simulink model "full_model"  (R2021a)
settings: Solver=VariableStepAuto  StartTime=0.0  StopTime=50  RelTol=1e-3
values from neighbouring files (symbols this model uses):
  P = [real(P), imag(P)]    [black_pz.m]    (also in black_rlocus.m; black_rlocus_fine.m)
  R = rlocus(sys)    [black_rlocus.m]    (also in black_rlocus_fine.m = rlocus(sys,k))
undefined symbols (not defined in the file or in its folder): A_rocket, alpha_fine, Alt_sequence, Ang_max, Baro_exp, cm_fine, cm_lookup, Ct_rot, D, drag_lookup, drag_rot_lookup, drag_wave_lookup, g, h_0, I_s, I_x_lookup, I_yz_lookup, L_b, lift_lookup, lift_rot_lookup, m_burn, M_crit, M_fine, m_prop_max, m_wet, N, P_0, Phi, Pos_sequence, Psi, Q, r_E, S_e, T_b, T_lookup, T_max, T_max_s, t_P, t_S, t_V, Theta, Tilt_max, Ts_hev, Ts_hor, U, Upsilon, V, v_land, W
settings Model: Creator=EpEp  LastModifiedBy=EpEp
settings DebuggingCC: UnderSpecifiedDimensionMsg=warning

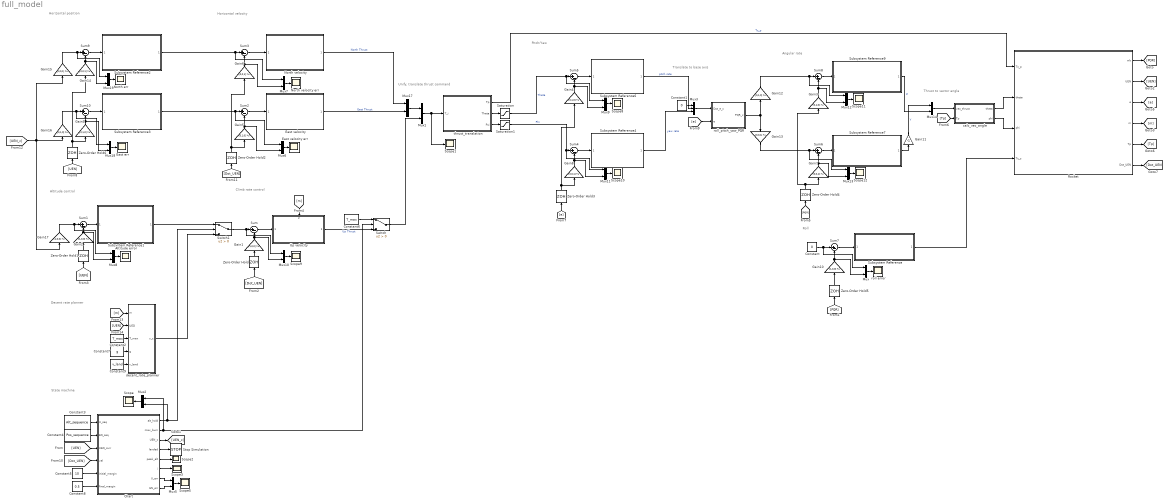
== system full_model ==
  note: Decent rate planner
  note: State machine
  note: Thrust to vector angle
  note: Roll
  note: Angular rate
  note: Translate to base axis
  note: Unify, translate thrust command
  note: Pitch/Yaw
  note: Climb rate control
  note: Altitude control
  note: Horizontal velocity
  note: Horizontal position
  Altitude error : Scope
  Chart : Stateflow chart  TreatAsAtomicUnit=on
  Constant : Constant  Value=0
  Constant1 : Constant  Value=0
  Constant2 : Constant  Value=T_max
  Constant3 : Constant  Value=Alt_sequence
  Constant4 : Constant  Value=Pos_sequence
  Constant5 : Constant  Value=10
  Constant6 : Constant  Value=T_max
  Constant7 : Constant  Value=g
  Constant8 : Constant  Value=0.5
  Constant9 : Constant  Value=v_land
  East err : Scope
  East velocity : Subsystem  ReferencedSubsystem=hor_vel_control
  East velocity err : Scope
  Gain{1..2,10,17} (4 alike) : Gain  Gain=[1,0,0]  Multiplication=Matrix(K*u)
  Gain11 : Gain  Gain=-1
  Gain{3..5,9,12,16} (6 alike) : Gain  Gain=[0,1,0]  Multiplication=Matrix(K*u)
  Gain{6..8,13..15} (6 alike) : Gain  Gain=[0,0,1]  Multiplication=Matrix(K*u)
  Mux{,1..2,5..14,17..19} (16 alike) : Mux  Inputs=2
  Mux3 : Mux  Inputs=3
  North err : Scope
  North velocity : Subsystem  ReferencedSubsystem=hor_vel_control
  North velocity err : Scope
  Rocket : Subsystem
  Saturation : Saturate  UpperLimit=Tilt_max  LowerLimit=-Tilt_max
  Saturation1 : Saturate  UpperLimit=Tilt_max  LowerLimit=-Tilt_max
  Scope{,1..3,5,8..12} (10 alike) : Scope
  Stop Simulation : Stop
  Subsystem Reference : Subsystem  ReferencedSubsystem=roll_controller
  Subsystem Reference1 : Subsystem  ReferencedSubsystem=alt_control
  Subsystem Reference2 : Subsystem  ReferencedSubsystem=pos_controller
  Subsystem Reference3 : Subsystem  ReferencedSubsystem=pos_controller
  Subsystem Reference4 : Subsystem  ReferencedSubsystem=ang_control
  Subsystem Reference6 : Subsystem  ReferencedSubsystem=ang_control
  Subsystem Reference7 : Subsystem  ReferencedSubsystem=rate_controller
  Subsystem Reference9 : Subsystem  ReferencedSubsystem=rate_controller
  Sum{,1..10} (11 alike) : Sum  Inputs=|+-
  Switch : Switch  Criteria=u2 > Threshold
  Switch1 : Switch  Criteria=u2 > Threshold
  Up velocity : Subsystem  ReferencedSubsystem=climb_control_PI
      settings: PortSchema="{\"entries\":[{\"content\":{\"sides\":[{\"content\":{\"connectorIds\":[\"In1\"]},\"type\":\"ConnectorPlacement.EquallySpacedRectSide\",\"uuid\":\"95254302-9a74-4c7f-a882-67c73735b286\"},{\"content\":{\"connectorIds\":[\"Out1\"],\"side\":\"RIGHT\"},\"type\":\"ConnectorPlacement.EquallySpacedRectSide\",\"uuid\":\"514a7716-605a-484c-b4b8-fcaa29f8a508\"},{\"content\":{\"connectorIds\":[\"In2\"],\"side\":\"TOP\"},\"type\":\"ConnectorPlacement.EquallySpacedRectSide\",\"uuid\":\"a977e3e4-e86d-439d-b6e9-39df081e30dd\"}]},\"type\":\"ConnectorPlacement.EquallySpacedConnector\",\"uuid\":\"b9474d80-c721-4f49-b50c-8544c213d6ea\"}],\"packageUris\":[\"http://schema.mathworks.com/mf0/Connector/R2020b\"],\"version\":\"1.0\"}"
  Zero-Order Hold : ZeroOrderHold  SampleTime=Ts_hev
  Zero-Order Hold1 : ZeroOrderHold  SampleTime=Ts_hev
  Zero-Order Hold{2..6} (5 alike) : ZeroOrderHold  SampleTime=Ts_hor
  calc_vec_angle : MATLAB Function  TreatAsAtomicUnit=on
  decent_rate_planner : MATLAB Function  TreatAsAtomicUnit=on
  roll error : Scope
  roll_pitch_yaw_PQR : MATLAB Function  TreatAsAtomicUnit=on
  thrust_translation : MATLAB Function  TreatAsAtomicUnit=on
  wires:
  Rocket/1(wb) -> [PQR]
  Rocket/2(UEN) -> [UEN]
  Gain1/1 -> Mux10/2, Sum/2
  [Dot_UEN] -> Zero-Order Hold/1
  Sum/1 -> Up velocity/1
  Sum1/1 -> Subsystem Reference1/1
  Gain2/1 -> Mux8/2, Sum1/2
  Rocket/4(m) -> [m]
  [m] -> Up velocity/2
  Subsystem Reference6/1 -> Mux3/2  "pitch rate"
  Sum8/1 -> Subsystem Reference9/1
  Gain3/1 -> Sum8/2, Mux12/2
  Rocket/3(e) -> [e]
  Gain4/1 -> Sum5/2, Mux9/2
  Sum5/1 -> Subsystem Reference6/1
  Sum2/1 -> East velocity/1
  Gain5/1 -> Sum2/2, Mux6/2
  Rocket/5(Tp) -> [Tp]
  East velocity/1 -> Mux17/2  "East Thrust"
  Zero-Order Hold2/1 -> Gain6/1, Gain5/1
  Sum3/1 -> North velocity/1
  Gain6/1 -> Mux7/2, Sum3/2
  North velocity/1 -> Mux17/1  "North Thrust"
  thrust_translation/1(Tp) -> Rocket/1(Tc_p)  "Tc_p"
  Subsystem Reference4/1 -> Mux3/3  "yaw rate"
  Gain8/1 -> Sum4/2, Mux11/2
  Gain7/1 -> Sum6/2, Mux13/2
  Sum4/1 -> Subsystem Reference4/1
  Sum6/1 -> Subsystem Reference7/1
  Zero-Order Hold4/1 -> Gain7/1, Gain3/1
  thrust_translation/2(Theta) -> Saturation/1
  thrust_translation/3(Psi) -> Saturation1/1
  Saturation/1 -> Sum5/1, Mux9/1  "Theta"
  Saturation1/1 -> Mux11/1, Sum4/1  "Phi"
  Subsystem Reference7/1 -> Gain11/1
  Zero-Order Hold/1 -> Gain1/1
  [UEN] -> Zero-Order Hold1/1
  Zero-Order Hold1/1 -> Gain2/1
  [Dot_UEN] -> Zero-Order Hold2/1
  [e] -> Zero-Order Hold3/1
  [PQR] -> Zero-Order Hold4/1
  Mux6/1 -> East velocity err/1
  Mux7/1 -> North velocity err/1
  Mux8/1 -> Altitude error/1
  Mux10/1 -> Scope9/1
  Mux9/1 -> Scope8/1
  Mux11/1 -> Scope10/1
  Mux12/1 -> Scope11/1
  Mux13/1 -> Scope12/1
  calc_vec_angle/2(phi) -> Rocket/3(phi)
  Mux1/1 -> Scope1/1, thrust_translation/1(T_i)
  Mux17/1 -> Mux1/1
  Subsystem Reference/1 -> Rocket/4(Tc_s)
  [PQR] -> Zero-Order Hold5/1
  Zero-Order Hold5/1 -> Gain10/1
  Gain10/1 -> Mux/2, Sum7/2
  Sum7/1 -> Subsystem Reference/1
  Constant/1 -> Mux/1, Sum7/1
  Mux/1 -> roll error/1
  calc_vec_angle/1(theta) -> Rocket/2(theta)
  Subsystem Reference9/1 -> Mux14/2  "Z"
  Gain11/1 -> Mux14/1  "Y"
  Mux14/1 -> calc_vec_angle/1(vec_thrust)
  [Tp] -> calc_vec_angle/2(Tp)
  Constant1/1 -> Mux3/1
  [e] -> roll_pitch_yaw_PQR/2(e)
  Mux3/1 -> roll_pitch_yaw_PQR/1(Dot_e_c)
  roll_pitch_yaw_PQR/1(PQR_c) -> Gain12/1, Gain13/1
  Gain12/1 -> Mux12/1, Sum8/1
  Gain13/1 -> Mux13/1, Sum6/1
  Constant3/1 -> Chart/1(U_seq)
  Constant4/1 -> Chart/2(EN_seq)
  Sum9/1 -> Subsystem Reference2/1
  Sum10/1 -> Subsystem Reference3/1
  Gain9/1 -> Mux18/2, Sum10/2
  [UEN] -> Zero-Order Hold6/1
  Zero-Order Hold6/1 -> Gain14/1, Gain9/1
  Gain14/1 -> Mux19/2, Sum9/2
  Mux18/1 -> East err/1
  Mux19/1 -> North err/1
  Zero-Order Hold3/1 -> Gain4/1, Gain8/1
  Rocket/6(Dot_UEN) -> [Dot_UEN]
  Subsystem Reference2/1 -> Mux7/1, Sum3/1
  Subsystem Reference3/1 -> Mux6/1, Sum2/1
  [UEN] -> Chart/3(UEN_curr)
  Constant5/1 -> Chart/5(initial_margin)
  Chart/4(landed) -> Stop Simulation/1
  Chart/1(alt_hold) -> Mux2/2, Switch1/2
  Switch1/1 -> Mux10/1, Sum/1
  Subsystem Reference1/1 -> Switch1/1
  Chart/2(max_burn) -> Mux2/1, Switch/2
  Mux2/1 -> Scope/1
  Constant6/1 -> Switch/1
  Switch/1 -> Mux1/2
  Up velocity/1 -> Switch/3  "Up Thrust"
  [Dot_UEN] -> Chart/4(vel)
  Chart/5(peak_alt) -> Scope2/1
  Constant8/1 -> Chart/6(final_margin)
  Chart/6(i) -> Scope3/1
  Chart/7(U_err) -> Mux5/1
  Chart/8(EN_err) -> Mux5/2
  Mux5/1 -> Scope5/1
  Chart/3(UEN_c) -> [UEN_c]
  Gain15/1 -> Mux19/1, Sum9/1
  Gain16/1 -> Mux18/1, Sum10/1
  [UEN_c] -> Gain17/1, Gain16/1, Gain15/1
  Gain17/1 -> Mux8/1, Sum1/1
  decent_rate_planner/1(v_c) -> Switch1/3
  [m] -> decent_rate_planner/1(m)
  Constant2/1 -> decent_rate_planner/3(T_max)
  Constant7/1 -> decent_rate_planner/4(g)
  Constant9/1 -> decent_rate_planner/5(v_land)
  [UEN] -> decent_rate_planner/2(UED)

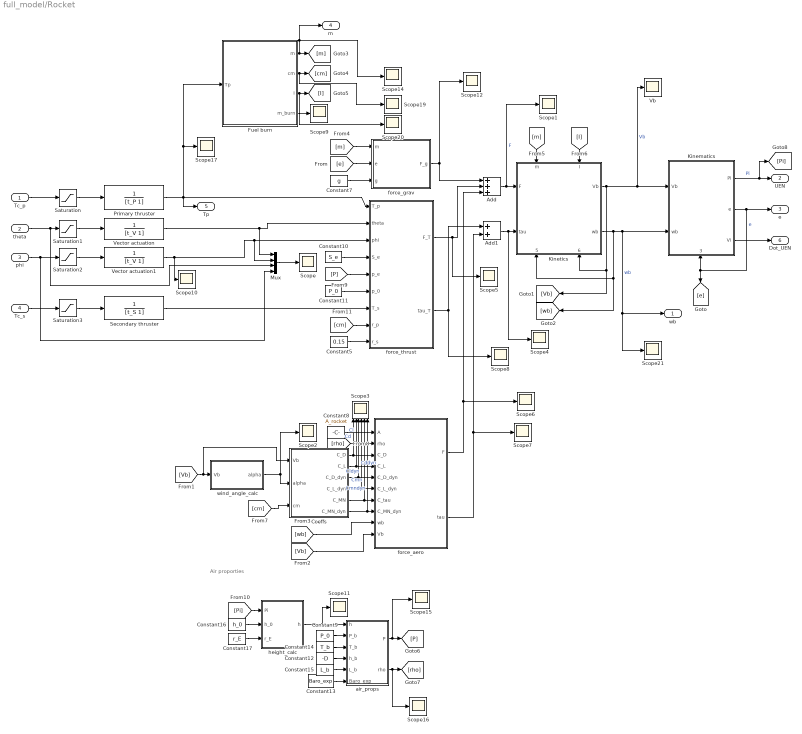
== system full_model/Rocket ==
  note: Air proporties
  Tc_p : Inport
  theta : Inport  Port=2
  phi : Inport  Port=3
  Tc_s : Inport  Port=4
  Add : Sum  Inputs=+++
  Add1 : Sum
  Coeffs : Subsystem
  Constant10 : Constant  Value=S_e
  Constant11 : Constant  Value=P_0
  Constant12 : Constant  Value=-D
  Constant13 : Constant  Value=Baro_exp
  Constant14 : Constant  Value=T_b
  Constant15 : Constant  Value=L_b
  Constant16 : Constant  Value=h_0
  Constant17 : Constant  Value=r_E
  Constant5 : Constant  Value=0.15
  Constant7 : Constant  Value=g
  Constant8 : Constant  Value=A_rocket
  Constant9 : Constant  Value=P_0
  Fuel burn : Subsystem
  Kinematics : Subsystem
      settings: PortSchema="{\"entries\":[{\"content\":{\"sides\":[{\"content\":{\"connectorIds\":[\"In1\",\"In2\"]},\"type\":\"ConnectorPlacement.EquallySpacedRectSide\",\"uuid\":\"eae29983-0cae-4ee4-868d-1c50a6f3cfea\"},{\"content\":{\"connectorIds\":[\"Out1\",\"Out2\",\"Out3\"],\"side\":\"RIGHT\"},\"type\":\"ConnectorPlacement.EquallySpacedRectSide\",\"uuid\":\"bdc65933-6547-4251-8b39-00a552207d7f\"},{\"content\":{\"connectorIds\":[],\"side\":\"TOP\"},\"type\":\"ConnectorPlacement.EquallySpacedRectSide\",\"uuid\":\"ee33c1e0-7d1f-4e43-84a0-58639e27ac5c\"},{\"content\":{\"connectorIds\":[\"In3\"],\"side\":\"BOTTOM\"},\"type\":\"ConnectorPlacement.EquallySpacedRectSide\",\"uuid\":\"b7ff67e5-658b-4688-8b54-a193f9f6d197\"}]},\"type\":\"ConnectorPlacement.EquallySpacedConnector\",\"uuid\":\"f4d120fb-b3cd-4fc8-b600-b4efda2a2057\"}],\"packageUris\":[\"http://schema.mathworks.com/mf0/Connector/R2020b\"],\"version\":\"1.0\"}"
  Kinetics : Subsystem
      settings: PortSchema="{\"entries\":[{\"content\":{\"sides\":[{\"content\":{\"connectorIds\":[\"In1\",\"In2\"]},\"type\":\"ConnectorPlacement.EquallySpacedRectSide\",\"uuid\":\"44e96cf1-b775-4685-9d80-77fe5197a3b8\"},{\"content\":{\"connectorIds\":[\"Out1\",\"Out2\"],\"side\":\"RIGHT\"},\"type\":\"ConnectorPlacement.EquallySpacedRectSide\",\"uuid\":\"1ce02f86-3039-4a72-8110-79d6c21885aa\"},{\"content\":{\"connectorIds\":[\"In3\",\"In4\"],\"side\":\"TOP\"},\"type\":\"ConnectorPlacement.EquallySpacedRectSide\",\"uuid\":\"c3c088af-4572-4447-8e34-ea7d8079d91e\"},{\"content\":{\"connectorIds\":[\"In5\",\"In6\"],\"side\":\"BOTTOM\"},\"type\":\"ConnectorPlacement.EquallySpacedRectSide\",\"uuid\":\"9c91a776-c86a-41f9-9dfe-00178419c6d9\"}]},\"type\":\"ConnectorPlacement.EquallySpacedConnector\",\"uuid\":\"6fbd1051-4f47-4787-a689-54b5a6d8998f\"}],\"packageUris\":[\"http://schema.mathworks.com/mf0/Connector/R2020b\"],\"version\":\"1.0\"}"
  Mux : Mux
  Primary thruster : TransferFcn  Denominator=[t_P 1]
  Saturation : Saturate  UpperLimit=T_max  LowerLimit=0
  Saturation1 : Saturate  UpperLimit=Ang_max  LowerLimit=-Ang_max
  Saturation2 : Saturate  UpperLimit=Ang_max  LowerLimit=-Ang_max
  Saturation3 : Saturate  UpperLimit=T_max_s  LowerLimit=-T_max_s
  Scope{,1..2,4..12,14..17,19..21} (19 alike) : Scope
  Scope3 : Scope  NumInputPorts=6
  Secondary thruster : TransferFcn  Denominator=[t_S 1]
  Vb : Scope
  Vector actuation : TransferFcn  Denominator=[t_V 1]
  Vector actuation1 : TransferFcn  Denominator=[t_V 1]
  air_props : MATLAB Function  TreatAsAtomicUnit=on
  force_aero : MATLAB Function  TreatAsAtomicUnit=on
  force_grav : MATLAB Function  TreatAsAtomicUnit=on
  force_thrust : MATLAB Function  TreatAsAtomicUnit=on
  height_calc : MATLAB Function  TreatAsAtomicUnit=on
  wind_angle_calc : MATLAB Function  TreatAsAtomicUnit=on
  wb : Outport
  UEN : Outport  Port=2
  e : Outport  Port=3
  m : Outport  Port=4
  Tp : Outport  Port=5
  Dot_UEN : Outport  Port=6
  wires:
  Primary thruster/1 -> force_thrust/1(T_p), Tp/1, Fuel burn/1(Tp), Scope17/1
  [Vb] -> Coeffs/1(Vb), wind_angle_calc/1(Vb)
  Fuel burn/1(m) -> Scope14/1, m/1, [m]
  Kinetics/2(wb) -> [wb], Kinetics/5(5), Scope21/1, wb/1, Kinematics/2(wb)  "wb"
  force_grav/1(F_g) -> Scope12/1, Add/1
  force_aero/2(tau) -> Scope7/1, Add1/2
  Kinematics/1(Pi) -> [Pi], UEN/1  "Pi"
  Kinematics/2(e) -> e/1, Kinematics/3(3), [e]  "e"
  Kinetics/1(Vb) -> [Vb], Kinetics/6(6), Vb/1, Kinematics/1(Vb)  "Vb"
  air_props/2(rho) -> Scope16/1, [rho]
  Coeffs/3(C_D_dyn) -> Scope3/3, force_aero/5(C_D_dyn)  "Cddyn"
  height_calc/1(h) -> Scope11/1, air_props/1(h)
  [cm] -> force_thrust/8(r_p)
  Add/1 -> Scope1/1, Kinetics/1(F)  "F"
  Coeffs/2(C_L) -> Scope3/2, force_aero/4(C_L)  "Cl"
  Add1/1 -> Scope4/1, Kinetics/2(tau)
  Coeffs/4(C_L_dyn) -> Scope3/4, force_aero/6(C_L_dyn)  "Cldyn"
  Coeffs/5(C_MN) -> Scope3/5, force_aero/7(C_tau)  "Cmn"
  Constant9/1 -> air_props/2(P_b)
  force_thrust/2(tau_T) -> Scope8/1, Add1/1
  Coeffs/1(C_D) -> Scope3/1, force_aero/3(C_D)  "Cd"
  air_props/1(P) -> Scope15/1, [P]
  [Pi] -> height_calc/1(Pi)
  Constant14/1 -> air_props/3(T_b)
  Coeffs/6(C_MN_dyn) -> Scope3/6, force_aero/8(C_MN_dyn)  "Cmndyn"
  Constant5/1 -> force_thrust/9(r_s)
  Constant7/1 -> force_grav/3(g)
  wind_angle_calc/1(alpha) -> Scope2/1, Coeffs/2(alpha)
  [I] -> Kinetics/4(I)
  Constant16/1 -> height_calc/2(h_0)
  Constant11/1 -> force_thrust/6(p_0)
  Fuel burn/4(m_burn) -> Scope9/1
  [e] -> force_grav/2(e)
  Secondary thruster/1 -> force_thrust/7(T_s)
  [m] -> force_grav/1(m)
  Constant13/1 -> air_props/6(Baro_exp)
  [m] -> Kinetics/3(m)
  force_aero/1(F) -> Add/3, Scope6/1
  force_thrust/1(F_T) -> Scope5/1, Add/2
  [rho] -> force_aero/2(rho)
  [P] -> force_thrust/5(p_e)
  Constant12/1 -> air_props/4(h_b)
  Constant15/1 -> air_props/5(L_b)
  Constant8/1 -> force_aero/1(A)
  [wb] -> force_aero/9(wb)
  Constant10/1 -> force_thrust/4(S_e)
  Constant17/1 -> height_calc/3(r_E)
  Fuel burn/3(I) -> Scope20/1, [I]
  [cm] -> Coeffs/3(cm)
  Fuel burn/2(cm) -> Scope19/1, [cm]
  [Vb] -> force_aero/10(Vb)
  Vector actuation/1 -> Mux/1, force_thrust/2(theta)
  Vector actuation1/1 -> Scope10/1, Mux/2, force_thrust/3(phi)
  Kinematics/3(Vi) -> Dot_UEN/1
  Saturation/1 -> Primary thruster/1
  Tc_p/1 -> Saturation/1
  Saturation1/1 -> Vector actuation/1
  theta/1 -> Mux/3, Saturation1/1
  Saturation2/1 -> Vector actuation1/1
  phi/1 -> Mux/4, Saturation2/1
  Saturation3/1 -> Secondary thruster/1
  Tc_s/1 -> Saturation3/1
  Mux/1 -> Scope/1

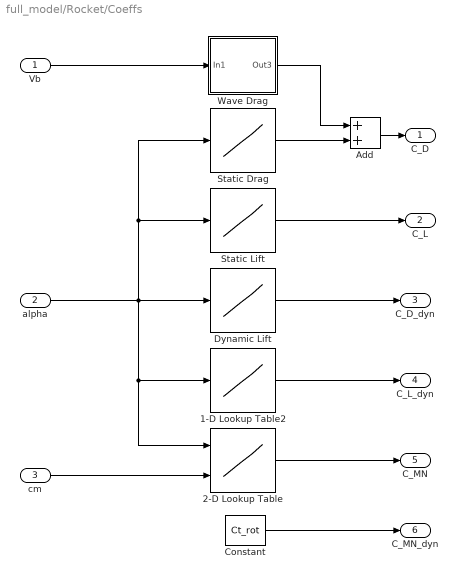
== system full_model/Rocket/Coeffs ==
  Vb : Inport
  alpha : Inport  Port=2
  cm : Inport  Port=3
  1-D Lookup Table2 : Lookup_n-D  NumberOfTableDimensions=1  BreakpointsForDimension1=alpha_fine  Table=lift_rot_lookup  InternalRulePriority=Speed  RndMeth=Simplest  InputSameDT=on
  2-D Lookup Table : Lookup_n-D  BreakpointsForDimension1=alpha_fine  BreakpointsForDimension2=cm_fine  Table=T_lookup  InternalRulePriority=Speed  RndMeth=Simplest  InputSameDT=on
      settings: InputPortMap=u0,u1
  Add : Sum
  Constant : Constant  Value=Ct_rot
  Dynamic Lift : Lookup_n-D  NumberOfTableDimensions=1  BreakpointsForDimension1=alpha_fine  Table=drag_rot_lookup  InternalRulePriority=Speed  RndMeth=Simplest  InputSameDT=on
  Static Drag : Lookup_n-D  NumberOfTableDimensions=1  BreakpointsForDimension1=alpha_fine  Table=drag_lookup  InternalRulePriority=Speed  RndMeth=Simplest  InputSameDT=on
  Static Lift : Lookup_n-D  NumberOfTableDimensions=1  BreakpointsForDimension1=alpha_fine  Table=lift_lookup  InternalRulePriority=Speed  RndMeth=Simplest  InputSameDT=on
  Wave Drag : Subsystem
  C_D : Outport
  C_L : Outport  Port=2
  C_D_dyn : Outport  Port=3
  C_L_dyn : Outport  Port=4
  C_MN : Outport  Port=5
  C_MN_dyn : Outport  Port=6
  wires:
  alpha/1 -> Static Drag/1, Static Lift/1, 2-D Lookup Table/1, 1-D Lookup Table2/1, Dynamic Lift/1
  cm/1 -> 2-D Lookup Table/2
  Static Lift/1 -> C_L/1
  Dynamic Lift/1 -> C_D_dyn/1
  1-D Lookup Table2/1 -> C_L_dyn/1
  2-D Lookup Table/1 -> C_MN/1
  Constant/1 -> C_MN_dyn/1
  Static Drag/1 -> Add/2
  Vb/1 -> Wave Drag/1(In1)
  Wave Drag/1(Out3) -> Add/1
  Add/1 -> C_D/1

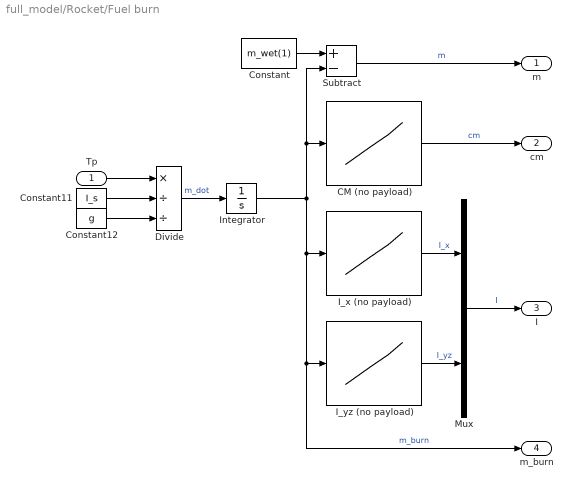
== system full_model/Rocket/Fuel burn ==
  Tp : Inport
  CM (no payload) : Lookup_n-D  NumberOfTableDimensions=1  BreakpointsForDimension1=[0,m_prop_max*2]  Table=cm_lookup  InternalRulePriority=Speed  RndMeth=Simplest  InputSameDT=on
  Constant : Constant  Value=m_wet(1)
  Constant11 : Constant  Value=I_s
  Constant12 : Constant  Value=g
  Divide : Product  Inputs=*//
  I_x (no payload) : Lookup_n-D  NumberOfTableDimensions=1  BreakpointsForDimension1=[0,m_prop_max*2]  Table=I_x_lookup  InternalRulePriority=Speed  RndMeth=Simplest  InputSameDT=on
  I_yz (no payload) : Lookup_n-D  NumberOfTableDimensions=1  BreakpointsForDimension1=m_burn*2  Table=I_yz_lookup  InternalRulePriority=Speed  RndMeth=Simplest  InputSameDT=on
  Integrator : Integrator
  Mux : Mux  Inputs=2
  Subtract : Sum  Inputs=+-
  m : Outport
  cm : Outport  Port=2
  I : Outport  Port=3
  m_burn : Outport  Port=4
  wires:
  Divide/1 -> Integrator/1  "m_dot"
  Constant11/1 -> Divide/2
  Integrator/1 -> m_burn/1, I_yz (no payload)/1, I_x (no payload)/1, Subtract/2, CM (no payload)/1  "m_burn"
  Tp/1 -> Divide/1
  Constant/1 -> Subtract/1
  Subtract/1 -> m/1  "m"
  CM (no payload)/1 -> cm/1  "cm"
  I_x (no payload)/1 -> Mux/1  "I_x"
  I_yz (no payload)/1 -> Mux/2  "I_yz"
  Mux/1 -> I/1  "I"
  Constant12/1 -> Divide/3

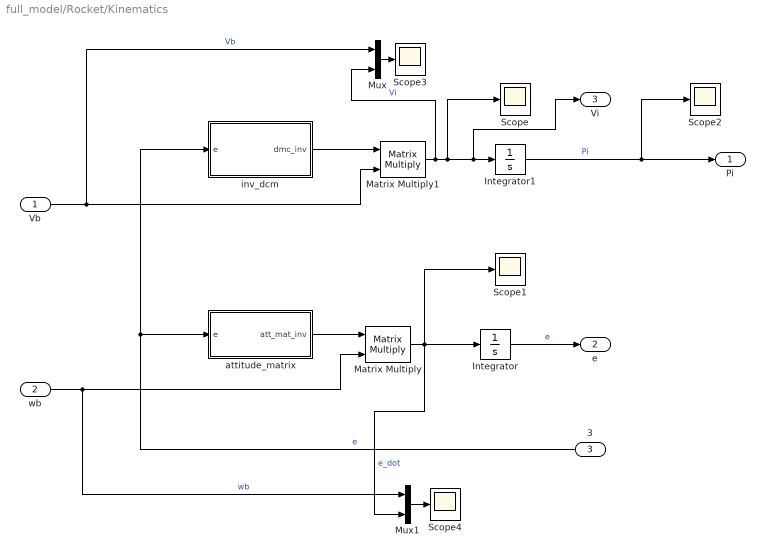
== system full_model/Rocket/Kinematics ==
  Vb : Inport
  wb : Inport  Port=2
  3 : Inport  Port=3
  Integrator : Integrator  InitialCondition=[Phi;Theta;Psi]
  Integrator1 : Integrator  InitialCondition=[Upsilon;E;N]  LimitOutput=on  LowerSaturationLimit=-[0;inf;inf]
  Matrix Multiply : Product  Multiplication=Matrix(*)
  Matrix Multiply1 : Product  Multiplication=Matrix(*)
  Mux : Mux  Inputs=2
  Mux1 : Mux  Inputs=2
  Scope{,1..4} (5 alike) : Scope
  attitude_matrix : MATLAB Function  TreatAsAtomicUnit=on
  inv_dcm : MATLAB Function  TreatAsAtomicUnit=on
  Pi : Outport
  e : Outport  Port=2
  Vi : Outport  Port=3
  wires:
  attitude_matrix/1(att_mat_inv) -> Matrix Multiply/1
  wb/1 -> Mux1/1, Matrix Multiply/2  "wb"
  Matrix Multiply/1 -> Scope1/1, Mux1/2, Integrator/1  "e_dot"
  Integrator/1 -> e/1  "e"
  inv_dcm/1(dmc_inv) -> Matrix Multiply1/1
  Vb/1 -> Mux/1, Matrix Multiply1/2  "Vb"
  Matrix Multiply1/1 -> Mux/2, Scope/1, Vi/1, Integrator1/1  "Vi"
  3/1 -> inv_dcm/1(e), attitude_matrix/1(e)  "e"
  Integrator1/1 -> Scope2/1, Pi/1  "Pi"
  Mux/1 -> Scope3/1
  Mux1/1 -> Scope4/1

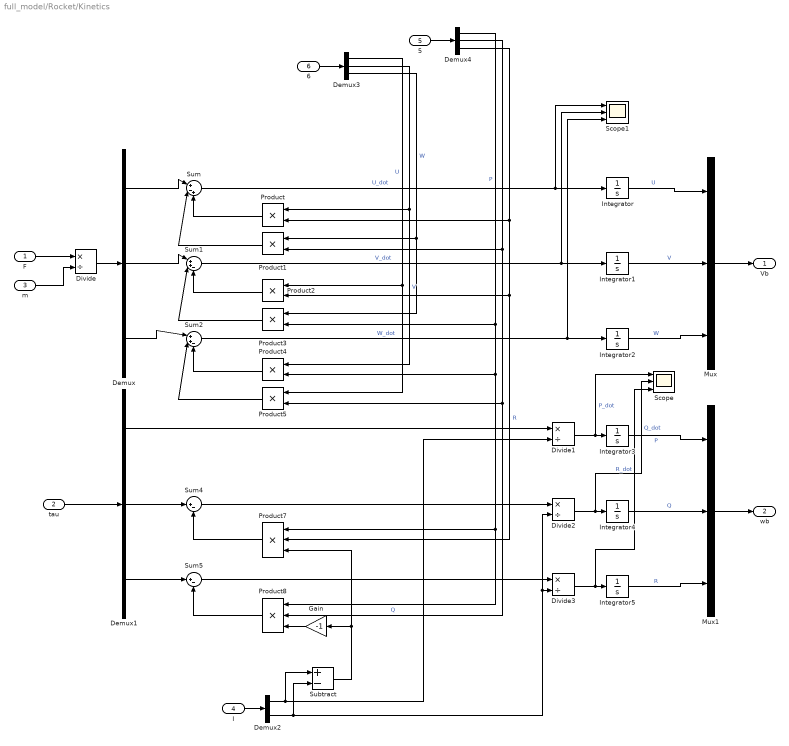
== system full_model/Rocket/Kinetics ==
  F : Inport  PortDimensions=[3,1]
  tau : Inport  Port=2  PortDimensions=[3,1]
  m : Inport  Port=3
  I : Inport  Port=4
  5 : Inport  Port=5
  6 : Inport  Port=6
  Demux{,1,3..4} (4 alike) : Demux  Outputs=3
  Demux2 : Demux  Outputs=2
  Divide{,1..3} (4 alike) : Product  Inputs=*/
  Gain : Gain  Gain=-1
  Integrator : Integrator  InitialCondition=U
  Integrator1 : Integrator  InitialCondition=V
  Integrator2 : Integrator  InitialCondition=W
  Integrator3 : Integrator  InitialCondition=P
  Integrator4 : Integrator  InitialCondition=Q
  Integrator5 : Integrator  InitialCondition=R
  Mux : Mux  Inputs=3
  Mux1 : Mux  Inputs=3
  Product{,1..5} (6 alike) : Product
  Product7 : Product  Inputs=3
  Product8 : Product  Inputs=3
  Scope : Scope  NumInputPorts=3
  Scope1 : Scope  NumInputPorts=3
  Subtract : Sum  Inputs=+-
  Sum : Sum  Inputs=|+-+
  Sum1 : Sum  Inputs=|++-
  Sum2 : Sum  Inputs=|++-
  Sum4 : Sum  Inputs=|+-
  Sum5 : Sum  Inputs=|+-
  Vb : Outport  PortDimensions=[3,1]
  wb : Outport  Port=2  PortDimensions=[3,1]
  wires:
  Demux/1 -> Sum/1
  Demux1/3 -> Sum5/1
  Demux/2 -> Sum1/1
  Demux/3 -> Sum2/1
  Demux1/2 -> Sum4/1
  Product1/1 -> Sum/2
  Product/1 -> Sum/3
  Product3/1 -> Sum1/2
  Product2/1 -> Sum1/3
  Product4/1 -> Sum2/3
  Product5/1 -> Sum2/2
  F/1 -> Divide/1
  Divide/1 -> Demux/1
  m/1 -> Divide/2
  tau/1 -> Demux1/1
  Product7/1 -> Sum4/2
  Product8/1 -> Sum5/2
  Demux1/1 -> Divide1/1
  Divide1/1 -> Scope/1, Integrator3/1  "P_dot"
  Sum/1 -> Scope1/1, Integrator/1  "U_dot"
  Sum1/1 -> Scope1/2, Integrator1/1  "V_dot"
  Sum2/1 -> Scope1/3, Integrator2/1  "W_dot"
  I/1 -> Demux2/1
  Demux2/1 -> Divide1/2, Subtract/1
  Divide2/1 -> Scope/2, Integrator4/1  "Q_dot"
  Divide3/1 -> Scope/3, Integrator5/1  "R_dot"
  Sum5/1 -> Divide3/1
  Sum4/1 -> Divide2/1
  Demux2/2 -> Divide3/2, Divide2/2, Subtract/2
  Subtract/1 -> Product7/3, Gain/1
  Gain/1 -> Product8/3
  6/1 -> Demux3/1
  5/1 -> Demux4/1
  Demux3/2 -> Product4/1, Product/1  "V"
  Demux4/3 -> Product7/2, Product2/2, Product/2  "R"
  Demux3/3 -> Product3/1, Product1/1  "W"
  Demux4/1 -> Product3/2, Product8/1, Product7/1, Product4/2  "P"
  Demux3/1 -> Product5/1, Product2/1  "U"
  Demux4/2 -> Product1/2, Product5/2, Product8/2  "Q"
  Integrator/1 -> Mux/1  "U"
  Integrator2/1 -> Mux/3  "W"
  Integrator1/1 -> Mux/2  "V"
  Mux/1 -> Vb/1
  Integrator5/1 -> Mux1/3  "R"
  Integrator4/1 -> Mux1/2  "Q"
  Integrator3/1 -> Mux1/1  "P"
  Mux1/1 -> wb/1

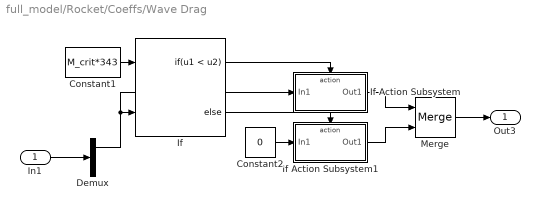
== system full_model/Rocket/Coeffs/Wave Drag ==
  In1 : Inport
  Constant1 : Constant  Value=M_crit*343
  Constant2 : Constant  Value=0
  Demux : Demux  Outputs=3
  If : If  NumInputs=2  IfExpression=u1 < u2
  If Action Subsystem : Subsystem  TreatAsAtomicUnit=on
  If Action Subsystem1 : Subsystem  TreatAsAtomicUnit=on
  Merge : Merge
  Out3 : Outport
  wires:
  Merge/1 -> Out3/1
  If/2 -> If Action Subsystem1/Action
  Demux/1 -> If/2, If Action Subsystem/1(In1)
  If Action Subsystem1/1(Out1) -> Merge/2
  Constant1/1 -> If/1
  If Action Subsystem/1(Out1) -> Merge/1
  If/1 -> If Action Subsystem/Action
  Constant2/1 -> If Action Subsystem1/1(In1)
  In1/1 -> Demux/1

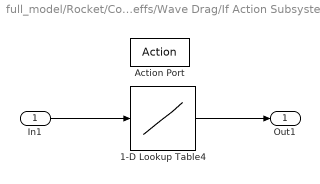
== system full_model/Rocket/Coeffs/Wave Drag/If Action Subsystem ==
  In1 : Inport
  Action Port : ActionPort  ActionPortLabel=if(u1 < u2)
  1-D Lookup Table4 : Lookup_n-D  NumberOfTableDimensions=1  BreakpointsForDimension1=M_fine*343  Table=drag_wave_lookup  InternalRulePriority=Speed  RndMeth=Simplest  InputSameDT=on
  Out1 : Outport
  wires:
  In1/1 -> 1-D Lookup Table4/1
  1-D Lookup Table4/1 -> Out1/1

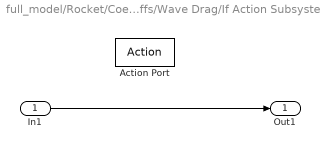
== system full_model/Rocket/Coeffs/Wave Drag/If Action Subsystem1 ==
  In1 : Inport
  Action Port : ActionPort  ActionPortLabel=else
  Out1 : Outport
  wires:
  In1/1 -> Out1/1

== matlab function full_model/Rocket/force_thrust ==
  data: T_p input; theta input; phi input; S_e input; p_e input; p_0 input; F_T output; T_s input; r_p input; r_s input; tau_T output
function [F_T, tau_T] = fcn(T_p,theta, phi,S_e,p_e,p_0, T_s, r_p, r_s)
    if T_p ~= 0
        T_p = T_p + S_e*(p_0-p_e);
    end
    F_dir = [cos(theta)*cos(phi); 
             sin(phi); 
             -sin(theta)];
    F_T = F_dir*T_p;
    tau_T = [T_s*r_s; 
             F_T(3)*r_p; 
             -F_T(2)*r_p];

== matlab function full_model/Rocket/force_grav ==
  data: m input; F_g output; e input; g input
function F_g = fcn(m,e,g)
    Phi = e(1);
    Theta = e(2);
    Psi = e(3);
    grav_mat = [-cos(Psi)*cos(Theta);
                -cos(Psi)*sin(Theta)*sin(Phi) + sin(Psi)*cos(Phi);
                -cos(Psi)*sin(Theta)*cos(Phi) - sin(Psi)*sin(Phi)];
    F_g = grav_mat*m*g;

== matlab function full_model/Rocket/Kinematics/attitude_matrix ==
  data: att_mat_inv output; e input
function att_mat_inv = fcn(e)
    Phi = e(1);
    Theta = e(2);
%     att_mat = [1    , sin(Phi)*tan(Theta)   , cos(Phi)*tan(Theta)   ;
%                0    , cos(Phi)              , -sin(Phi)             ;
%                0    , sin(Phi)*sec(Theta)   , cos(Phi)*sec(Theta)   ;];
           
    att_mat_inv = [1,    sin(Phi)*tan(Theta),  cos(Phi)*tan(Theta);
                    0,              cos(Phi),            -sin(Phi);
                    0,   sin(Phi)*sec(Theta), cos(Phi)*sec(Theta)];

== matlab function full_model/Rocket/Kinematics/inv_dcm ==
  data: e input; dmc_inv output
function dmc_inv = fcn(e)
    Phi = e(1);
    Theta = e(2);
    Psi = e(3);
    
    dmc_inv = [cos(Psi)*cos(Theta), cos(Psi)*sin(Theta)*sin(Phi) - sin(Psi)*cos(Phi), cos(Psi)*sin(Theta)*cos(Phi) + sin(Psi)*sin(Phi);
               sin(Psi)*cos(Theta), sin(Psi)*sin(Theta)*sin(Phi) + cos(Psi)*cos(Phi), sin(Psi)*sin(Theta)*cos(Phi) - cos(Psi)*sin(Phi);
                       -sin(Theta),                              cos(Theta)*sin(Phi),                              cos(Theta)*cos(Phi)];

== matlab function full_model/Rocket/force_aero ==
  data: A input; rho input; C_D input; F output; tau output; C_L input; C_D_dyn input; C_L_dyn input; C_tau input; C_MN_dyn input; wb input; Vb input
function [F,tau] = fcn(A,rho,C_D,C_L,C_D_dyn,C_L_dyn,C_tau,C_MN_dyn,wb,Vb)
    Vb_norm_sqr = Vb'*Vb;
    % Get unit velocity vector
    if Vb_norm_sqr ~= 0
        Vb_unit = Vb/sqrt(Vb_norm_sqr);
    else
        Vb_unit = Vb;
    end
    
    % Get unit force vectors
    Drag_vec = -Vb_unit;
    Torque_vec = cross(Vb_unit,[1;0;0]);
    Lift_vec = cross(Torque_vec,Vb_unit);
    
    C_XYZ = Drag_vec*C_D + Lift_vec*C_L;
    C_LMN = Torque_vec*C_tau;
    
    F = 0.5*rho*A*Vb_norm_sqr*C_XYZ;
    tau = 0.5*rho*A*Vb_norm_sqr*C_LMN;

== matlab function full_model/Rocket/wind_angle_calc ==
  data: Vb input; alpha output
function alpha  = fcn(Vb)
    Vb_norm = sqrt(Vb'*Vb);
    if Vb_norm ~= 0
        alpha = acos(dot(Vb/Vb_norm,[1;0;0]));
    else
        alpha = 0;
    end

== matlab function full_model/Rocket/air_props ==
  data: h input; P output; rho output; P_b input; T_b input; h_b input; L_b input; Baro_exp input
function [P,rho] = fcn(h,P_b,T_b,h_b,L_b,Baro_exp)
    T = T_b+(h-h_b)*L_b;
    P = P_b*(T/T_b)^Baro_exp;
    rho = (P*0.02897)/(8.3145*T);

== matlab function full_model/Rocket/height_calc ==
  data: Pi input; h output; h_0 input; r_E input
function h = fcn(Pi,h_0,r_E)
    h = sqrt(Pi(1)^2+Pi(2)^2+(r_E+h_0+Pi(3))^2)-r_E;

== matlab function full_model/thrust_translation ==
  data: T_i input; Tp output; Theta output; Psi output
function [Tp,Theta,Psi] = fcn(T_i)
    if T_i(3) > 0
        Tp = sqrt(T_i'*T_i);
        Psi = atan(T_i(2)/(T_i(3)));
        Theta = -atan(T_i(1)/sqrt(T_i(1)*T_i(1)+T_i(3)*T_i(3)));
    else
        Tp = 0;
        Psi = 0;
        Theta = 0;
    end

== stateflow chart full_model/Chart ==
  state Control_states [parallel]
    settings: executionOrder=1
    state Launch_pad
    state Max_burn
      en:
      max_burn = 1;
    state Hold_altitude
      du:
      alt_hold = 1;
    state Constant_decent
    (default) -> Launch_pad
    Launch_pad -> Hold_altitude [order 2] : [launch &&...
        | abs(U_err) <= initial_margin]
    Launch_pad -> Max_burn [order 1] : [launch &&...
        | abs(U_err) > initial_margin]
    (junction 30) -> Max_burn [order 2] : [peak_alt - U_seq(i) < 0]
    Max_burn -> Hold_altitude : [abs(peak_alt - U_seq(i)) < initial_margin]...
        | {max_burn = 0;}
    Hold_altitude -> (junction 30) : [abs(peak_alt - U_seq(i)) > initial_margin]...
        | {alt_hold = 0;}
    Constant_decent -> Hold_altitude : [~landing &&...
        | abs(peak_alt - U_seq(i)) < initial_margin]
    (junction 30) -> Constant_decent [order 1] : [peak_alt - U_seq(i) > 0]
  state Waypoint_follow [parallel]
    settings: executionOrder=2
    state First_waypoint
      en:
      g = 9.81;
      i = 1;
      seq_len = length(U_seq);
      U_err = U_seq(i) - UEN_curr(3);
      EN_err = EN_seq(:,i) - UEN_curr(1:2);
      peak_alt = (vel(1)*vel(1))/(2*g)+UEN_curr(1);
      Control_states.launch
    state Current_waypoint
      en,du:
      UEN_c = [U_seq(i);EN_seq(:,i)];
      U_err = U_seq(i) - UEN_curr(1);
      EN_err = EN_seq(:,i) - UEN_curr(2:3);
      peak_alt = (vel(1)*vel(1))/(2*g)+UEN_curr(1);
    state Next_waypoint
      en:
      i = i + 1;
    state Landing
      du:
      Control_states.landing
    state Landed
      landed = 1;
    (default) -> First_waypoint
    First_waypoint -> Current_waypoint
    Next_waypoint -> Current_waypoint [order 2]
    Current_waypoint -> Next_waypoint : [abs(U_err) < final_margin &&...
        | abs(EN_err(1)) < final_margin &&...
        | abs(EN_err(2)) < final_margin]
    Next_waypoint -> Landing [order 1] : [i == seq_len]
    Landing -> Landed : [abs(UEN_curr(1)-U_seq(seq_len)) < 0.01]
  data: U_seq input; EN_seq input; seq_len local; UEN_curr input; vel input; initial_margin input; alt_hold output; max_burn output; UEN_c output; landed output; g local; peak_alt output; final_margin input; i output; U_err output; EN_err output
  events: landing local FUNCTION_CALL_EVENT; launch local FUNCTION_CALL_EVENT

== matlab function full_model/calc_vec_angle ==
  data: vec_thrust input; theta output; Tp input; phi output
function [theta, phi] = fcn(vec_thrust, Tp)
    if vec_thrust(1) >= Tp
        phi = pi;
    elseif vec_thrust(1) <= -Tp
        phi = -pi;
    else
        phi = asin(vec_thrust(1)/Tp);
    end
    
    if vec_thrust(2) >= Tp
        theta = -pi;
    elseif vec_thrust(2) <= -Tp
        theta = pi;
    else
        theta = -asin(vec_thrust(2)/Tp);
    end

== matlab function full_model/decent_rate_planner ==
  data: m input; UED input; T_max input; v_c output; g input; v_land input
function v_c = fcn(m,UED,T_max,g,v_land)
    a_max = T_max/m-g;
    alt = UED(1);
    v_c = (3*v_land-sqrt(9*v_land^2-8*(v_land^2-alt*a_max)))/4;

== matlab function full_model/roll_pitch_yaw_PQR ==
  data: Dot_e_c input; PQR_c output; e input
function PQR_c = fcn(Dot_e_c, e)
    Phi = e(1);
    Theta = e(2);

    att_mat = [ 1,        0,          -sin(Theta);
                0, cos(Phi),  sin(Phi)*cos(Theta);
                0, -sin(Phi),  cos(Phi)*cos(Theta);];
    PQR_c = att_mat*Dot_e_c;
